simulink subsystem "BatteryStatus"  (R2024a)
settings: Solver=VariableStepAuto  StartTime=0.0  StopTime=10.0  RelTol=1e-3
libraries: uavmavlinklib x1
settings Model: Creator=gurt1  LastModifiedBy=gurt1

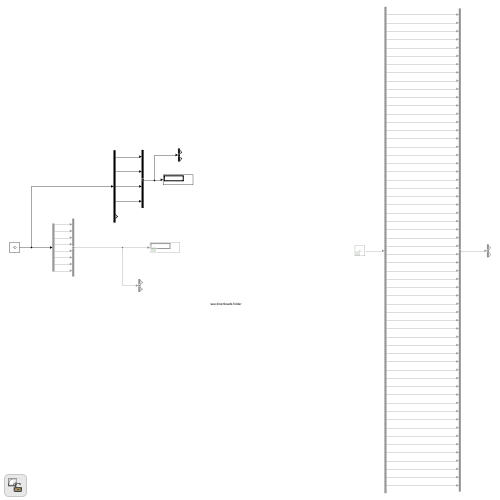
[thumbnail: Simulink's stored preview of the top-level diagram]
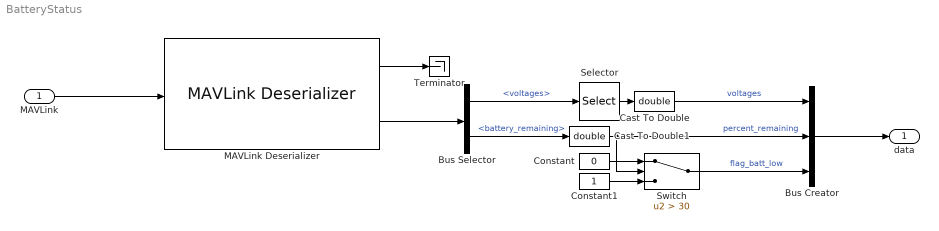
== system BatteryStatus ==
  MAVLink : Inport
  Bus Creator : BusCreator  Inputs=3
  Bus Selector : BusSelector  OutputSignals=Payload.voltages,Payload.battery_remaining
  Cast To Double : DataTypeConversion  OutDataTypeStr=double  SaturateOnIntegerOverflow=off  RndMeth=Floor
  Cast To Double1 : DataTypeConversion  OutDataTypeStr=double  SaturateOnIntegerOverflow=off  RndMeth=Floor
  Constant : Constant  Value=0
  Constant1 : Constant
  MAVLink Deserializer : uavmavlinklib/MAVLink Deserializer  dialectSource=Select from standard MAVLink dialects  dialect=common.xml  dialectCustom=common.xml  version=2  messageType=BATTERY_STATUS  inputDataLength=off  SystemIDFilter=off  systemID=1  ComponentIDFilter=off  componentID=1  queueMsg=off  queueMsgSize=50  dropNum=off
  Selector : Selector  InputPortWidth=10  IndexOptions=Index vector (dialog)  Indices=[1]  OutputSizes=1
  Switch : Switch  Criteria=u2 > Threshold  Threshold=30  SaturateOnIntegerOverflow=off  InputSameDT=off
  Terminator : Terminator
  data : Outport
  wires:
  MAVLink/1 -> MAVLink Deserializer/1
  MAVLink Deserializer/1 -> Terminator/1
  MAVLink Deserializer/2 -> Bus Selector/1
  Bus Creator/1 -> data/1
  Bus Selector/1 -> Selector/1  "<voltages>"
  Bus Selector/2 -> Cast To Double1/1  "<battery_remaining>"
  Cast To Double1/1 -> Bus Creator/2, Switch/2  "percent_remaining"
  Cast To Double/1 -> Bus Creator/1  "voltages"
  Selector/1 -> Cast To Double/1
  Switch/1 -> Bus Creator/3  "flag_batt_low"
  Constant/1 -> Switch/1
  Constant1/1 -> Switch/3
